simulink model "BicycleModelAccel"  (R2021a)
settings: Solver=VariableStepAuto  StartTime=0.0  StopTime=10.0  RelTol=1e-3
settings Model: Creator=Pratham  LastModifiedBy=Pratham

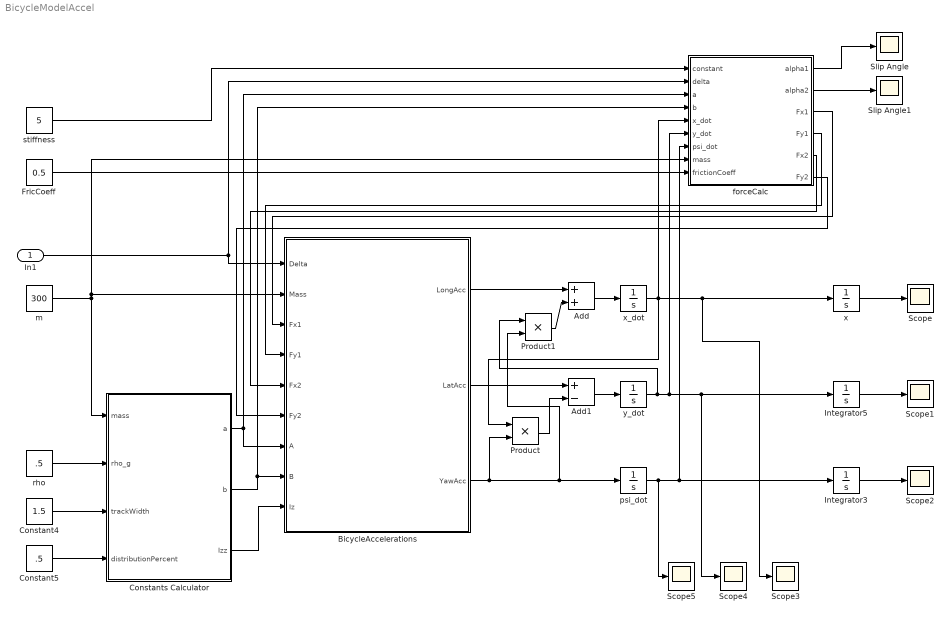
== system BicycleModelAccel ==
  In1 : Inport  OutMin=[0]  OutMax=[15]
  Add : Sum
  Add1 : Sum  Inputs=+-
  BicycleAccelerations : MATLAB Function  TreatAsAtomicUnit=on
  Constant4 : Constant  Value=1.5
  Constant5 : Constant  Value=.5
  Constants Calculator : MATLAB Function  TreatAsAtomicUnit=on
  FricCoeff : Constant  Value=0.5
  Integrator3 : Integrator
  Integrator5 : Integrator
  Product : Product
  Product1 : Product
  Scope{,1..5} (6 alike) : Scope
  Slip Angle : Scope
  Slip Angle1 : Scope
  forceCalc : MATLAB Function  TreatAsAtomicUnit=on
  m : Constant  Value=300
  psi_dot : Integrator
  rho : Constant  Value=.5
  stiffness : Constant  Value=5
  x : Integrator
  x_dot : Integrator  InitialCondition=10
  y_dot : Integrator  InitialCondition=10
  wires:
  In1/1 -> forceCalc/2(delta), BicycleAccelerations/1(Delta)
  m/1 -> forceCalc/8(mass), BicycleAccelerations/2(Mass), Constants Calculator/1(mass)
  rho/1 -> Constants Calculator/2(rho_g)
  Constants Calculator/1(a) -> BicycleAccelerations/7(A), forceCalc/3(a)
  Constants Calculator/2(b) -> forceCalc/4(b), BicycleAccelerations/8(B)
  Constants Calculator/3(Izz) -> BicycleAccelerations/9(Iz)
  Constant4/1 -> Constants Calculator/3(trackWidth)
  Constant5/1 -> Constants Calculator/4(distributionPercent)
  Integrator3/1 -> Scope2/1
  Integrator5/1 -> Scope1/1
  psi_dot/1 -> forceCalc/7(psi_dot), Integrator3/1, Scope5/1
  forceCalc/3(Fx1) -> BicycleAccelerations/3(Fx1)
  forceCalc/4(Fy1) -> BicycleAccelerations/4(Fy1)
  forceCalc/1(alpha1) -> Slip Angle/1
  FricCoeff/1 -> forceCalc/9(frictionCoeff)
  stiffness/1 -> forceCalc/1(constant)
  x/1 -> Scope/1
  x_dot/1 -> forceCalc/5(x_dot), x/1, Scope3/1, Product/1
  BicycleAccelerations/3(YawAcc) -> Product1/2, psi_dot/1, Product/2
  Product1/1 -> Add/2
  BicycleAccelerations/1(LongAcc) -> Add/1
  Add/1 -> x_dot/1
  Add1/1 -> y_dot/1
  BicycleAccelerations/2(LatAcc) -> Add1/1
  Product/1 -> Add1/2
  y_dot/1 -> Product1/1, forceCalc/6(y_dot), Integrator5/1, Scope4/1
  forceCalc/6(Fy2) -> BicycleAccelerations/6(Fy2)
  forceCalc/5(Fx2) -> BicycleAccelerations/5(Fx2)
  forceCalc/2(alpha2) -> Slip Angle1/1

== matlab function BicycleModelAccel/Constants Calculator ==
  data: a output; b output; mass input; Izz output; rho_g input; trackWidth input; distributionPercent input
function [a, b, Izz] = constantCalcs(mass, rho_g, trackWidth, distributionPercent)
Izz = mass*(rho_g)^2;
a = trackWidth*distributionPercent;
b = trackWidth - a;
end

== matlab function BicycleModelAccel/BicycleAccelerations ==
  data: LongAcc output; LatAcc output; Delta input; Mass input; YawAcc output; Fx1 input size=2; Fy1 input size=2; Fx2 input; Fy2 input; A input; B input; Iz input
function [LongAcc, LatAcc, YawAcc] = BicycleAccelerations (Delta, Mass, ...
    Fx1, Fy1, Fx2, Fy2, A, B, Iz)

%% BA - Bicycle Accelerations Calculations
% 
% Inputs:
%  Delta   - (n,1 numeric) Lateral Acceleration        {y_ddot} [m/s^2]
%  Mass    - (n,1 numeric) Mass                        {m}      [kg]
%  Fx      - (n,2 numeric) Force X-Direction           {F_x}    [kg*m/s^2]
%  Fy      - (n,2 numeric) Force Y-Direction           {F_y}    [kg*m/s^2]
%  A       - (n,1 numeric) Length C.O.M to Front Tire  {lf}     [m]
%  B       - (n,1 numeric) Length C.O.M to Back Tire   {lb}     [m]
%  Iz      - (n,1 numeric) Yaw Moment of Inertia       {I_z}    [kg*m^2]
%
% Outputs:
%  LatAcc  - (n,1 numeric) Lateral Acceleration        {y_ddot} [m/s^2]
%  LongAcc - (n,1 numeric) Longitudinal Acceleration   {x_ddot} [m/s^2]
%  YawAcc  - (n,1 numeric) Yaw Acceleration            {x_dot}  [m/s]
%  
% Notes:
% N/A
%
% Author(s): 
% Pratham Goradia (prgoradia@ucdavis.edu) [Aug 2021 - Sep 2021] 

% Last Updated: 21-Sep-2021

%% Test Cases
if nargin == 0
    %%% Test Inputs
    Delta = 15; 
    
    Mass = 300; 
    A = 2;
    B = 3;
    
    Fx = [10, 10];
    Fy = [10,10];
    Iz = 5;
  
    
    fprintf('Executing Bicycle Accelerations() Test Cases: \n');
    
    
    [LongAcc, LatAcc, YawAcc] = BicycleAccelerations (Delta, Mass, Fx, Fy, A, B, Iz);
    
    
        
end
    
%% Computation

% Accelerations
LongAcc = (Fx1*cosd(Delta) - Fy1*sind(Delta) + Fx2)/Mass;
LatAcc = (Fy1*cosd(Delta) + Fx1*sind(Delta) + Fy2)/Mass;
YawAcc = (A*(Fy1*cosd(Delta) + Fx1*sind(Delta)) - B*Fy2)/Iz;
end

== matlab function BicycleModelAccel/forceCalc ==
  data: constant input; delta input; alpha1 output size=2; alpha2 output size=2; a input; b input; x_dot input; y_dot input; psi_dot input; Fx1 output; Fy1 output; mass input; frictionCoeff input; Fx2 output; Fy2 output
function [alpha1, alpha2, Fx1, Fy1, Fx2, Fy2]  = forceCalc(constant, delta, a, ... 
b, x_dot, y_dot, psi_dot, mass, frictionCoeff)
grav = 9.81;
Fx2 = 0;
Fy2 = 0;
alpha1 = delta - atand(y_dot + a.*psi_dot ./ x_dot);
alpha2 = -atand(y_dot - b.*psi_dot ./ x_dot);
Fx1 = constant.*alpha1 + mass.*grav.*frictionCoeff;
Fy1 = constant.*alpha2 + mass.*grav.*frictionCoeff;
end
